simulink model "Filtro_IIR_Butterworth_cuantizado"  (R2022a)
settings: Solver=ode4  StartTime=0.0  StopTime=Inf  FixedStep=1e-4  RelTol=1e-3  EnableMultiTasking=on
libraries: dsparch4 x1
settings Model: ExtModeTrigDuration=8  Creator=05983057  LastModifiedBy=05983057
settings OptimizationCC: DefaultUnderspecifiedDataType=single  EnhancedBackFolding=on  PassReuseOutputArgsAs=Individual arguments  MaxStackSize=1024  OptimizeBlockOrder=speed  DifferentSizesBufferReuse=on  OptimizationCustomize=off  DenormalBehavior=FlushToZero  EfficientTunableParamExpr=on
settings DebuggingCC: ParameterTunabilityLossMsg=error
settings HardwareCC: ProdBitPerChar=16  ProdBitPerInt=16  ProdBitPerPointer=32  ProdBitPerSizeT=32  ProdBitPerPtrDiffT=32  ProdLargestAtomicInteger=Integer  ProdLargestAtomicFloat=None  ProdWordSize=16  ProdLongLongMode=on  ProdHWDeviceType=Texas Instruments->C2000
settings SFSimCC: MATLABDynamicMemAlloc=off
settings RTWCC: SystemTargetFile=ert.tlc  HardwareBoard=TI Delfino F2833x  TemplateMakefile=ert_default_tmf  Toolchain=Texas Instruments Code Composer Studio (C2000)
settings CodeAppCC: ForceParamTrailComments=on  IgnoreCustomStorageClasses=off  OperatorAnnotations=on  SimulinkDataObjDesc=on  SFDataObjDesc=on  InsertBlockDesc=on
settings ERTTargetCC: CodeReplacementLibrary=TI C28x  ExtModeTransport=3

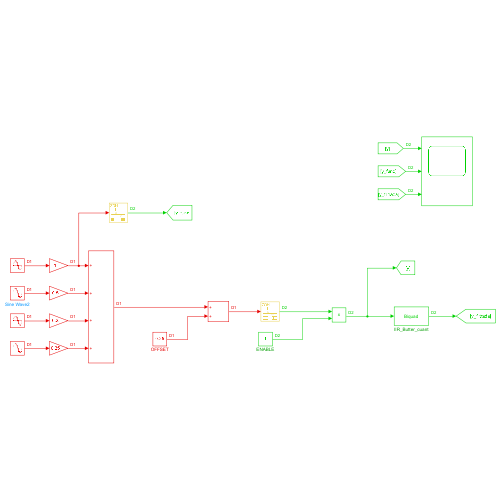
[thumbnail: Simulink's stored preview of the top-level diagram]
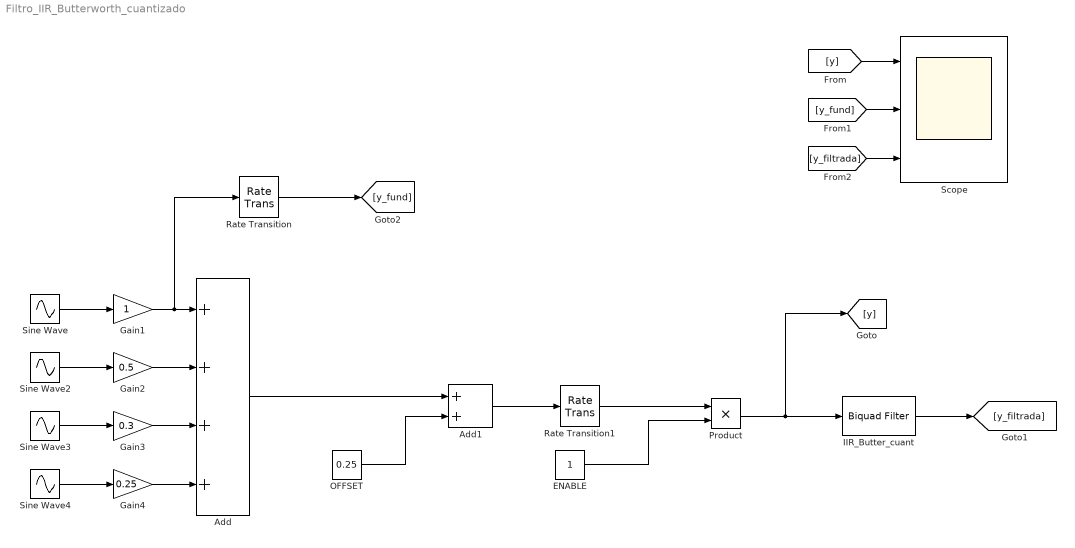
== system Filtro_IIR_Butterworth_cuantizado ==
  Add : Sum  Inputs=4
  Add1 : Sum  Inputs=2
  ENABLE : Constant  SampleTime=1e-3
  Gain1 : Gain
  Gain2 : Gain  Gain=0.5
  Gain3 : Gain  Gain=0.3
  Gain4 : Gain  Gain=0.25
  IIR_Butter_cuant : dsparch4/Biquad Filter  Tag=BlockMethodSubSystem  FilterSource=Dialog parameters  CoeffSource=Specify via dialog  FilterObject=BQF  IIRFiltStruct=Direct form II  BiQuadCoeffs=[1 0 -1 1 -1.70165482422892667 0.97142634017199625;1 0 -1 1 -1.9790904287308746 0.993203516439048806;1 0 -1 1 -1.65610305718772644 0.916929412589106319;1 0 -1 1 -1.96559918064114614 0.97970219354413679;1 0 -1 1 -1.61510576893720237 0.866129954344929009;1 0 -1 1 -1.95206530603725636 0.966244871002974626;1 0 -1 1 -1.57867138387322248 0.819168113953751331;1 0 -1 1 -1.93839221968360631 0.952737718294230373;1 0 -1 1 -1.54678221462388743 0.776137926416292756;1 0 -1 1 -1.92447748672752805 0.939083927215719649;1 0 -1 1 -1.51941093314976738 0.737105260904725723;1 0 -1 1 -1.91020869438995633 0.925180071518153069;1 0 -1 1 -1.49653538625661753 0.702124068928283385;1 0 -1 1 -1.8954582984307029 0.9109117694051454;1 0 -1 1 -1.88007680749597528 0.896148161979136271;1 0 -1 1 -1.47815284235453936 0.67125186756627786;1 0 -1 1 -1.86388332100344445 0.880734487412615064;1 0 -1 1 -1.46429507151041793 0.644565726675077166;1 0 -1 1 -1.84665182686570573 0.864481629425801645;1 0 -1 1 -1.45504622155860242 0.622180594471744008;1 0 -1 1 -1.82809058805132962 0.847150841159071355;1 0 -1 1 -1.45056647619208112 0.604272825921696732;1 0 -1 1 -1.80781004615104646 0.828430749944684575;1 0 -1 1 -1.45112632861610025 0.591113699440848794;1 0 -1 1 -1.78527148359753141 0.807902251678333738;1 0 -1 1 -1.45715944213078075 0.583121234336624661;1 0 -1 1 -1.75970460241081073 0.784986430654333156;1 0 -1 1 -1.4693461099900742 0.580944347487125756;1 0 -1 1 -1.72998543480201628 0.758881085287487211;1 0 -1 1 -1.48873603286410905 0.585597050333319769;1 0 -1 1 -1.69453565779751036 0.728568595178933132;1 0 -1 1 -1.51684944468755889 0.598618737393679767;1 0 -1 1 -1.65175047752190074 0.69337003674682085;1 0 -1 1 -1.55524949857546702 0.621883503643045121;1 0 -1 1 -1.60277052591023939 0.655402204254227239]  ScaleValues=[0.201996733587191085;0.201996733587191085;0.198548663624981025;0.198548663624981025;0.19531001654408553;0.19531001654408553;0.192286011881772495;0.192286011881772495;0.189479511792771588;0.189479511792771588;0.186891569840480415;0.186891569840480415;0.184521893477978732;0.184521893477978732;0.182369228605200023;0.182369228605200023;0.180431675681677006;0.180431675681677006;0.178706946947972622;0.178706946947972622;0.177192573766602163;0.177192573766602163;0.175886072215757916;0.175886072215757916;0.17478507404255475;0.17478507404255475;0.173887429023253159;0.173887429023253159;0.173191283753209385;0.173191283753209385;0.172695140932824648;0.172695140932824648;0.172397902339084669;0.172397902339084669;0.172298897872886408;1]  IC=0  ICnum=0  ICden=0  a0Flag=Warning  optimizeScaleValues=on  ScaleValueMode=Specify via input port (g)  InputProcessing=Columns as channels (frame based)  roundingMode=Floor  overflowMode=off  scaleValueFracLength=14  denProdOutputFracLength=30  denAccumFracLength=30  secondMemoryFracLength=15
  OFFSET : Constant  Value=0.25  SampleTime=1e-4
  Product : Product
  Rate Transition : RateTransition  OutPortSampleTime=1e-3
  Rate Transition1 : RateTransition  OutPortSampleTime=1e-3
  Scope : Scope  NumInputPorts=3
  Sine Wave : Sin  Frequency=50*2*pi  SampleTime=1e-4
  Sine Wave2 : Sin  Frequency=150*2*pi  SampleTime=1e-4
  Sine Wave3 : Sin  Amplitude=0.3  Frequency=250*2*pi  SampleTime=1e-4
  Sine Wave4 : Sin  Frequency=350*2*pi  SampleTime=1e-4
  wires:
  Add/1 -> Add1/1
  Sine Wave/1 -> Gain1/1
  Rate Transition1/1 -> Product/1
  Add1/1 -> Rate Transition1/1
  Sine Wave4/1 -> Gain4/1
  Sine Wave3/1 -> Gain3/1
  OFFSET/1 -> Add1/2
  Sine Wave2/1 -> Gain2/1
  Gain3/1 -> Add/3
  Gain1/1 -> Rate Transition/1, Add/1
  [y] -> Scope/1
  Gain4/1 -> Add/4
  ENABLE/1 -> Product/2
  Gain2/1 -> Add/2
  Product/1 -> IIR_Butter_cuant/1, [y]
  Rate Transition/1 -> [y_fund]
  [y_fund] -> Scope/2
  [y_filtrada] -> Scope/3
  IIR_Butter_cuant/1 -> [y_filtrada]
